simulink model "pendulum_model_2015a"  (R2015a)
settings: Solver=ode45  SolverMode=SingleTasking  StartTime=0  StopTime=10  MaxStep=.1  RelTol=1e-3  AbsTol=1e-6
values from neighbouring files (symbols this model uses):
  c = 0.0125    [PendulumExample.m]
  g = 9.81    [PendulumExample.m]
  len = 0.25    [PendulumExample.m]
  m = 4    [PendulumExample.m]
settings Model: CovHtmlReporting=off  ExtModeAutoUpdateStatusClock=off  Creator=The MathWorks, Inc.  LastModifiedBy=moham
settings DataIOCC: ExternalInput=[]  InitialState=[]  LimitDataPoints=off  SaveOutput=off  SaveTime=off
settings OptimizationCC: BlockReduction=off  BooleanDataType=off  InitFltsAndDblsToZero=on  BufferReusableBoundary=off
settings DebuggingCC: SaveWithParameterizedLinksMsg=none  SignalResolutionControl=TryResolveAllWithWarning  MultiTaskDSMMsg=warning  MultiTaskCondExecSysMsg=none  FcnCallInpInsideContextMsg=EnableAllAsWarning  BusObjectLabelMismatch=none
settings HardwareCC: TargetUnknown=on
settings GRTTargetCC: TargetFcnLib=ansi_tfl_tmw.mat  CombineOutputUpdateFcns=off  GRTInterface=on

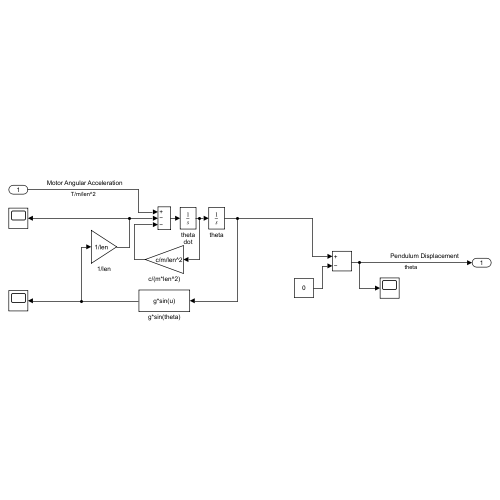
[thumbnail: Simulink's stored preview of the top-level diagram]
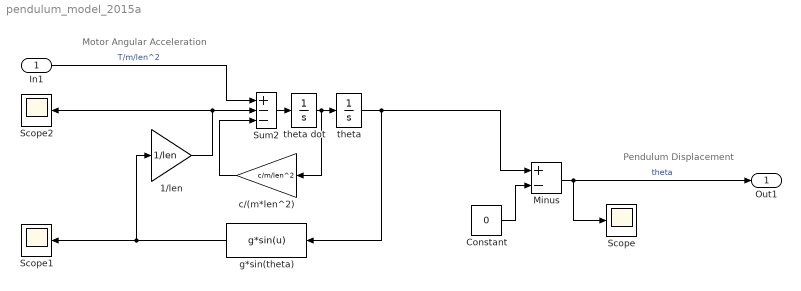
== system pendulum_model_2015a ==
  note: Pendulum Displacement
  note: Motor Angular Acceleration
  In1 : Inport
  1/len : Gain  Gain=1/len  SaturateOnIntegerOverflow=on  OutDataTypeStr=Inherit: Same as input  ParamDataTypeStr=Inherit: Same as input
  Constant : Constant  Value=0
  Minus : Sum  Inputs=+-
  Scope : Scope
      settings: TimeRange=auto  MaxDataPoints=5000  SaveToWorkspace=off  SaveName=ScopeData  YMin=-0.22137  YMax=1.9923  SampleTime=-1
  Scope1 : Scope
      settings: TimeRange=auto  MaxDataPoints=5000  SaveToWorkspace=off  YMin=-10.07693  YMax=10.38505  SampleTime=-1
  Scope2 : Scope
      settings: TimeRange=auto  MaxDataPoints=5000  SaveToWorkspace=off  SaveName=ScopeData2  YMin=-2.51923  YMax=2.59626  SampleTime=-1
  Sum2 : Sum  Inputs=+--  InputSameDT=on  SaturateOnIntegerOverflow=on  OutDataTypeStr=Inherit: Same as first input
  c/(m*len^2) : Gain  Gain=c/m/len^2  SaturateOnIntegerOverflow=on  OutDataTypeStr=Inherit: Same as input  ParamDataTypeStr=Inherit: Same as input
  g*sin(theta) : Fcn  Expr=g*sin(u)
  theta : Integrator  InitialCondition=1
  theta dot : Integrator
  Out1 : Outport
  wires:
  Sum2/1 -> theta dot/1
  c/(m*len^2)/1 -> Sum2/3
  theta dot/1 -> c/(m*len^2)/1, theta/1
  1/len/1 -> Scope2/1, Sum2/2
  g*sin(theta)/1 -> 1/len/1, Scope1/1
  In1/1 -> Sum2/1  "T/m/len^2"
  theta/1 -> Minus/1, g*sin(theta)/1
  Constant/1 -> Minus/2
  Minus/1 -> Scope/1, Out1/1  "theta"
